simulink model "project_file"  (R2023b)
settings: Solver=VariableStepAuto  StartTime=0.0  StopTime=30  MaxStep=0.1  RelTol=1e-3
model workspace (MAT data in the model file):
  Gradient = Simulink.Parameter
  Gradient.Value = 0
  Gradient.DataType = 'auto'
  Gradient.Complexity = 'real'
  Gradient.Dimensions = [1 1]
  Gravitational_Acceleration = Simulink.Parameter
  Gravitational_Acceleration.Value = 9.81
  Gravitational_Acceleration.DataType = 'auto'
  Gravitational_Acceleration.DocUnits = 'm/s^2'
  Gravitational_Acceleration.Complexity = 'real'
  Gravitational_Acceleration.Dimensions = [1 1]
  Kd = Simulink.Parameter
  Kd.Value = 0
  Kd.DataType = 'auto'
  Kd.Complexity = 'real'
  Kd.Dimensions = [1 1]
  Ki = Simulink.Parameter
  Ki.Value = 0.2
  Ki.DataType = 'auto'
  Ki.Complexity = 'real'
  Ki.Dimensions = [1 1]
  Kp = Simulink.Parameter
  Kp.Value = 0.9
  Kp.DataType = 'auto'
  Kp.Complexity = 'real'
  Kp.Dimensions = [1 1]
  Set_Speed = Simulink.Parameter
  Set_Speed.Value = 10
  Set_Speed.DataType = 'auto'
  Set_Speed.Complexity = 'real'
  Set_Speed.Dimensions = [1 1]
values from neighbouring files (symbols this model uses):
  gradient = 0    [post_credit_scene.m]    (also in simulink_link.m; simulink_part2_link.m = deg2rad(0))
  initial_speed = 0    [post_credit_scene.m]    (also in simulink_link.m; simulink_part2B_link.m; simulink_part2_link.m)
  Kd_m = 0    [post_credit_scene.m]    (also in simulink_link.m)
  Ki_m = 1.47    [post_credit_scene.m]    (also in simulink_link.m = 0.05)
  Kp_m = 1.81    [post_credit_scene.m]    (also in simulink_link.m = 0.05)
  linear_slope = (26.82) / zero_to_sixty    (= 3.08275862069)    [post_credit_scene.m]    (also in simulink_link.m = 3.44827586207; simulink_part2_link.m = 3.44827586207)
  max_speed = 30    [post_credit_scene.m]    (also in simulink_link.m; simulink_part2B_link.m = 60; simulink_part2_link.m)
libraries: simulink x1
settings Model: Creator=Matthew  LastModifiedBy=Matthew

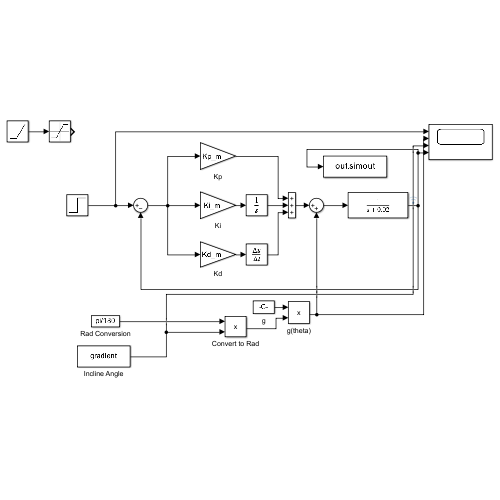
[thumbnail: Simulink's stored preview of the top-level diagram]
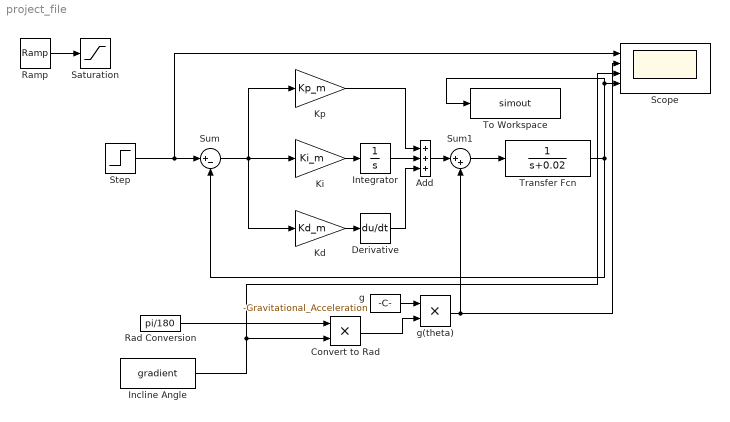
== system project_file ==
  Add : Sum  Inputs=+++
  Convert to Rad : Product
  Derivative : Derivative
  Incline Angle : Constant  Value=gradient
  Integrator : Integrator
  Kd : Gain  Gain=Kd_m
  Ki : Gain  Gain=Ki_m
  Kp : Gain  Gain=Kp_m
  Rad Conversion : Constant  Value=pi/180
  Ramp : simulink/Sources/Ramp  slope=linear_slope  start=0  InitialOutput=initial_speed  VectorParams1D=off
  Saturation : Saturate  UpperLimit=max_speed  LowerLimit=initial_speed
  Scope : Scope  NumInputPorts=4
  Step : Step  Time=10  Before=initial_speed  After=max_speed  SampleTime=0
  Sum : Sum  Inputs=|+-
  Sum1 : Sum  Inputs=|++
  To Workspace : ToWorkspace  VariableName=simout  SaveFormat=Timeseries  SampleTime=-1
  Transfer Fcn : TransferFcn  Denominator=[1 0.02]
  g : Constant  Value=-Gravitational_Acceleration
  g(theta) : Product
  wires:
  g(theta)/1 -> Sum1/2, Scope/2
  Sum1/1 -> Transfer Fcn/1
  Transfer Fcn/1 -> To Workspace/1, Scope/4, Sum/2
  Add/1 -> Sum1/1
  Kd/1 -> Derivative/1
  Derivative/1 -> Add/3
  Integrator/1 -> Add/2
  Sum/1 -> Kp/1, Ki/1, Kd/1
  Ki/1 -> Integrator/1
  Kp/1 -> Add/1
  Ramp/1 -> Saturation/1
  Incline Angle/1 -> Scope/3, Convert to Rad/2
  Convert to Rad/1 -> g(theta)/2
  g/1 -> g(theta)/1
  Rad Conversion/1 -> Convert to Rad/1
  Step/1 -> Scope/1, Sum/1
